simulink model "Lab_WiperSystem"  (R2024a)
settings: Solver=VariableStepDiscrete  StartTime=0.0  StopTime=10.0  MaxStep=1  RelTol=1e-3
libraries: simulink x5
settings Model: Creator=VICTUS  LastModifiedBy=VICTUS

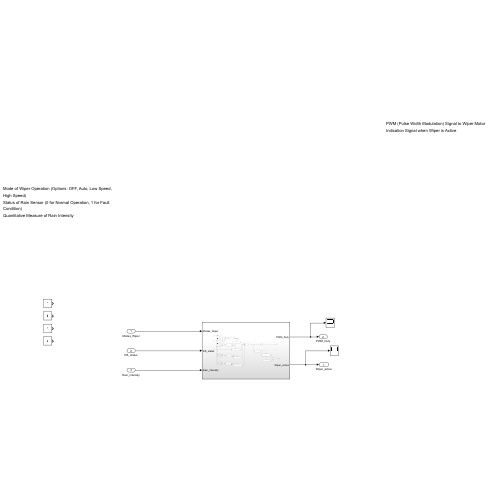
[thumbnail: Simulink's stored preview of the top-level diagram]
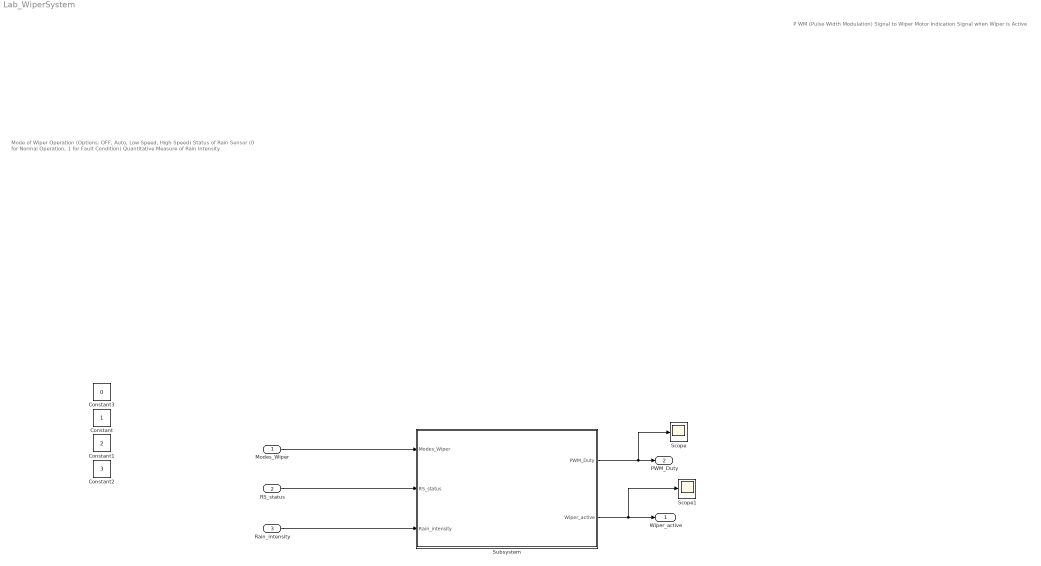
== system Lab_WiperSystem ==
  note: P WM (Pulse Width Modulation) Signal to Wiper Motor
      | Indication Signal when Wiper is Active
  note: Mode of Wiper Operation (Options: OFF, Auto, Low Speed, High Speed)
      | Status of Rain Sensor (0 for Normal Operation, 1 for Fault Condition)
      | Quantitative Measure of Rain Intensity
  Modes_Wiper : Inport
  RS_status : Inport  Port=2
  Rain_intensity : Inport  Port=3
  Constant : Constant
  Constant1 : Constant  Value=2
  Constant2 : Constant  Value=3
  Constant3 : Constant  Value=0
  Scope : Scope
  Scope1 : Scope
  Subsystem : Subsystem
  Wiper_active : Outport
  PWM_Duty : Outport  Port=2
  wires:
  Subsystem/1(PWM_Duty) -> Scope/1, PWM_Duty/1
  Subsystem/2(Wiper_active) -> Scope1/1, Wiper_active/1
  Modes_Wiper/1 -> Subsystem/1(Modes_Wiper)
  RS_status/1 -> Subsystem/2(RS_status)
  Rain_intensity/1 -> Subsystem/3(Rain_intensity)

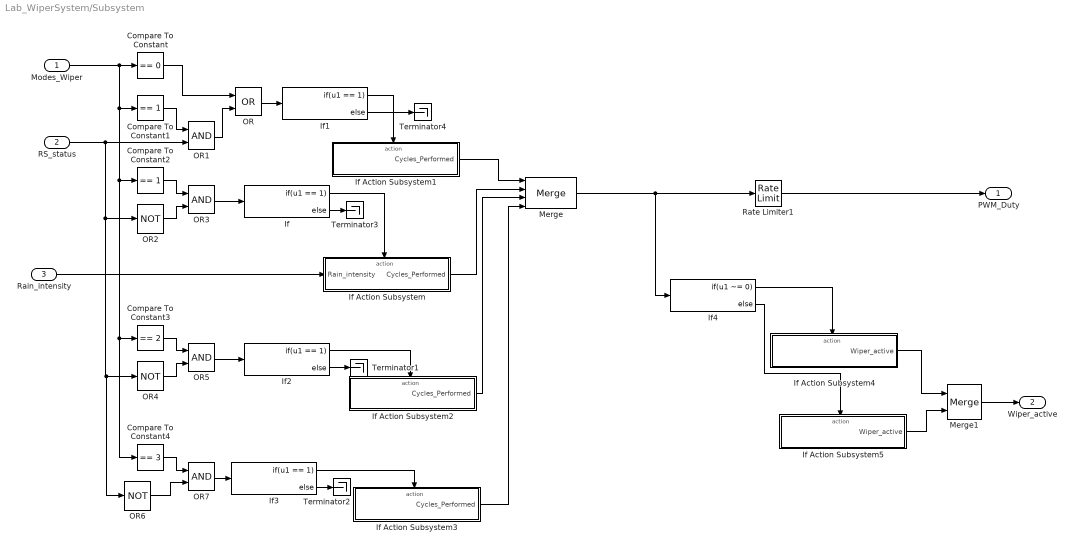
== system Lab_WiperSystem/Subsystem ==
  Modes_Wiper : Inport
  RS_status : Inport  Port=2
  Rain_intensity : Inport  Port=3
  Compare To Constant : simulink/Logic and Bit Operations/Compare To Constant  relop===  const=0  OutDataTypeStr=boolean
  Compare To Constant1 : simulink/Logic and Bit Operations/Compare To Constant  relop===  const=1  OutDataTypeStr=boolean
  Compare To Constant2 : simulink/Logic and Bit Operations/Compare To Constant  relop===  const=1  OutDataTypeStr=boolean
  Compare To Constant3 : simulink/Logic and Bit Operations/Compare To Constant  relop===  const=2  OutDataTypeStr=boolean
  Compare To Constant4 : simulink/Logic and Bit Operations/Compare To Constant  relop===  const=3  OutDataTypeStr=boolean
  If{,1..3} (4 alike) : If  IfExpression=u1 == 1
  If Action Subsystem : Subsystem  TreatAsAtomicUnit=on
  If Action Subsystem1 : Subsystem  TreatAsAtomicUnit=on
  If Action Subsystem2 : Subsystem  TreatAsAtomicUnit=on
  If Action Subsystem3 : Subsystem  TreatAsAtomicUnit=on
  If Action Subsystem4 : Subsystem  TreatAsAtomicUnit=on
  If Action Subsystem5 : Subsystem  TreatAsAtomicUnit=on
  If4 : If  IfExpression=u1 ~= 0
  Merge : Merge  Inputs=4
  Merge1 : Merge
  OR : Logic  Operator=OR  AllPortsSameDT=off  OutDataTypeStr=boolean
  OR{1,3,5,7} (4 alike) : Logic  AllPortsSameDT=off  OutDataTypeStr=boolean
  OR2 : Logic  Operator=NOT  AllPortsSameDT=off  OutDataTypeStr=boolean
  OR4 : Logic  Operator=NOT  AllPortsSameDT=off  OutDataTypeStr=boolean
  OR6 : Logic  Operator=NOT  AllPortsSameDT=off  OutDataTypeStr=boolean
  Rate Limiter1 : RateLimiter  RisingSlewLimit=0.1  FallingSlewLimit=-0.1  SampleTimeMode=inherited
  Terminator{1..4} (4 alike) : Terminator
  PWM_Duty : Outport
  Wiper_active : Outport  Port=2
  wires:
  If Action Subsystem1/1(Cycles_Performed) -> Merge/1
  RS_status/1 -> OR6/1, OR4/1, OR2/1, OR1/2
  OR1/1 -> OR/2
  If/1 -> If Action Subsystem/Action
  Modes_Wiper/1 -> Compare To Constant4/1, Compare To Constant3/1, Compare To Constant2/1, Compare To Constant1/1, Compare To Constant/1
  If1/1 -> If Action Subsystem1/Action
  Compare To Constant2/1 -> OR3/1
  OR4/1 -> OR5/2
  Compare To Constant/1 -> OR/1
  Rain_intensity/1 -> If Action Subsystem/1(Rain_intensity)
  If Action Subsystem3/1(Cycles_Performed) -> Merge/4
  If3/1 -> If Action Subsystem3/Action
  Compare To Constant3/1 -> OR5/1
  OR2/1 -> OR3/2
  Compare To Constant1/1 -> OR1/1
  OR/1 -> If1/1
  OR3/1 -> If/1
  If4/1 -> If Action Subsystem4/Action
  If2/1 -> If Action Subsystem2/Action
  If Action Subsystem2/1(Cycles_Performed) -> Merge/3
  If/2 -> Terminator3/1
  OR5/1 -> If2/1
  Compare To Constant4/1 -> OR7/1
  If2/2 -> Terminator1/1
  OR6/1 -> OR7/2
  OR7/1 -> If3/1
  If4/2 -> If Action Subsystem5/Action
  If3/2 -> Terminator2/1
  If1/2 -> Terminator4/1
  If Action Subsystem/1(Cycles_Performed) -> Merge/2
  If Action Subsystem4/1(Wiper_active) -> Merge1/1
  If Action Subsystem5/1(Wiper_active) -> Merge1/2
  Merge1/1 -> Wiper_active/1
  Merge/1 -> If4/1, Rate Limiter1/1
  Rate Limiter1/1 -> PWM_Duty/1

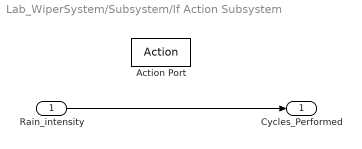
== system Lab_WiperSystem/Subsystem/If Action Subsystem ==
  Rain_intensity : Inport
  Action Port : ActionPort  ActionPortLabel=if(u1 == 1)
  Cycles_Performed : Outport
  wires:
  Rain_intensity/1 -> Cycles_Performed/1

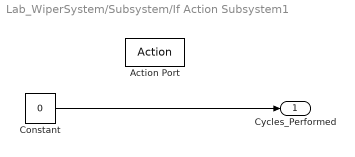
== system Lab_WiperSystem/Subsystem/If Action Subsystem1 ==
  Action Port : ActionPort  ActionPortLabel=if(u1 == 1)
  Constant : Constant  Value=0
  Cycles_Performed : Outport
  wires:
  Constant/1 -> Cycles_Performed/1

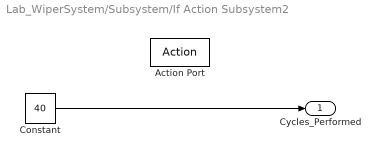
== system Lab_WiperSystem/Subsystem/If Action Subsystem2 ==
  Action Port : ActionPort  ActionPortLabel=if(u1 == 1)
  Constant : Constant  Value=40
  Cycles_Performed : Outport
  wires:
  Constant/1 -> Cycles_Performed/1

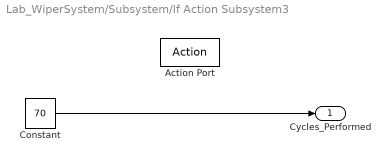
== system Lab_WiperSystem/Subsystem/If Action Subsystem3 ==
  Action Port : ActionPort  ActionPortLabel=if(u1 == 1)
  Constant : Constant  Value=70
  Cycles_Performed : Outport
  wires:
  Constant/1 -> Cycles_Performed/1

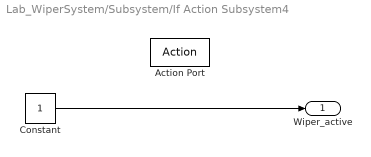
== system Lab_WiperSystem/Subsystem/If Action Subsystem4 ==
  Action Port : ActionPort  ActionPortLabel=if(u1 ~= 0)
  Constant : Constant
  Wiper_active : Outport
  wires:
  Constant/1 -> Wiper_active/1

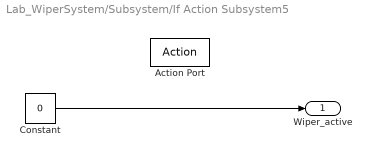
== system Lab_WiperSystem/Subsystem/If Action Subsystem5 ==
  Action Port : ActionPort  ActionPortLabel=else
  Constant : Constant  Value=0
  Wiper_active : Outport
  wires:
  Constant/1 -> Wiper_active/1
